simulink model "bike_model_yixiao"  (R2018b)
settings: Solver=FixedStepAuto  StartTime=0.0  StopTime=sim_time  FixedStep=Ts_IMU  MaxStep=Ts  RelTol=1e-3
undefined symbols (not defined in the file): A, A_kalman, B, b_compFilter, B_kalman, b_real, C, C_kalman, complementary, cumulative_dist_along_path, curvature, D, D_kalman, damp, Dead_Band, delay, direct_control, DiscIntNeverNeededParam, Discrete, DX, filter_model, forward_motor_dynamics, fr_oscil, g, gain, I_direct, I_lat, I_steer, IMU_height_model, IMU_height_real, initial_states, initial_x, initial_y, input_velocity, lambda_compFilter, lambda_real, lat_control, look_ahead, lqr_gains, max_handlebar, max_roll, max_steering_motor_acc, max_steering_motor_speed, min_handlebar, min_roll, min_steering_motor_acc, min_steering_motor_speed, Nc, noise, noise_acc, noise_encoder, noise_gyro, noise_hall, noise_pos_meas, Np, osc_roll, osc_steer, P_direct, P_lat, P_steer ... (+20)
libraries: simulink x14, mpclib x2, dspsigops x2, simulink_extras x1, ctrlSharedLib x1
(part 2 of 3)

== system bike_model_yixiao/Reference Position /Reference Position and Angle Selector ==
  total travelled distance : Inport
  1-D Lookup Table : Lookup_n-D  NumberOfTableDimensions=1  BreakpointsForDimension1=cumulative_dist_along_path  Table=path_x  ExtrapMethod=Clip  DiagnosticForOutOfRangeInput=Error  InternalRulePriority=Speed  RndMeth=Simplest  InputSameDT=on
  1-D Lookup Table1 : Lookup_n-D  NumberOfTableDimensions=1  BreakpointsForDimension1=cumulative_dist_along_path  Table=path_y  ExtrapMethod=Clip  DiagnosticForOutOfRangeInput=Error  InternalRulePriority=Speed  RndMeth=Simplest  InputSameDT=on
  Atan2 : Trigonometry  Operator=atan2
  Derivative : Derivative
  Derivative1 : Derivative
  Scope : Scope
  Unwrap : dspsigops/Unwrap  tol=pi  InputProcessing=Columns as channels (frame based)  running=off
  X_sigma : Outport
  Y_sigma : Outport  Port=2
  psi_sigma : Outport  Port=3
  wires:
  total travelled distance/1 -> 1-D Lookup Table1/1, 1-D Lookup Table/1
  Unwrap/1 -> Scope/1, psi_sigma/1
  1-D Lookup Table/1 -> X_sigma/1, Derivative1/1  "interpolated path x value"
  Derivative1/1 -> Atan2/2  "dx"
  Derivative/1 -> Atan2/1  "dy"
  Atan2/1 -> Unwrap/1
  1-D Lookup Table1/1 -> Y_sigma/1, Derivative/1  "interpolated path y value"

== system bike_model_yixiao/Reference Position /Subsystem1 ==
  total travelled distance : Inport
  1-D Lookup Table : Lookup_n-D  NumberOfTableDimensions=1  BreakpointsForDimension1=cumulative_dist_along_path  Table=path_x  ExtrapMethod=Clip  DiagnosticForOutOfRangeInput=Error  InternalRulePriority=Speed  RndMeth=Simplest  InputSameDT=on
  1-D Lookup Table1 : Lookup_n-D  NumberOfTableDimensions=1  BreakpointsForDimension1=cumulative_dist_along_path  Table=path_y  ExtrapMethod=Clip  DiagnosticForOutOfRangeInput=Error  InternalRulePriority=Speed  RndMeth=Simplest  InputSameDT=on
  Atan2 : Trigonometry  Operator=atan2
  Derivative : Derivative
  Derivative1 : Derivative
  Scope : Scope
  Unwrap : dspsigops/Unwrap  tol=pi  InputProcessing=Columns as channels (frame based)  running=off
  X_sigma : Outport
  Y_sigma : Outport  Port=2
  psi_sigma : Outport  Port=3
  wires:
  total travelled distance/1 -> 1-D Lookup Table1/1, 1-D Lookup Table/1
  Unwrap/1 -> Scope/1, psi_sigma/1
  1-D Lookup Table/1 -> X_sigma/1, Derivative1/1  "interpolated path x value"
  Derivative1/1 -> Atan2/2  "dx"
  Derivative/1 -> Atan2/1  "dy"
  Atan2/1 -> Unwrap/1
  1-D Lookup Table1/1 -> Y_sigma/1, Derivative/1  "interpolated path y value"

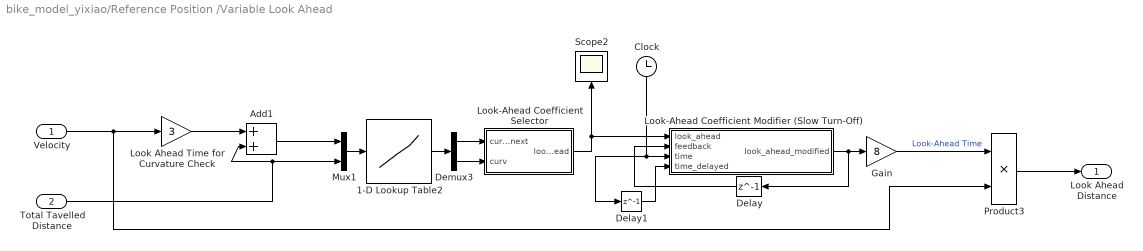
== system bike_model_yixiao/Reference Position /Variable Look Ahead ==
  Velocity : Inport
  Total Tavelled Distance : Inport  Port=2
  1-D Lookup Table2 : Lookup_n-D  NumberOfTableDimensions=1  BreakpointsForDimension1=cumulative_dist_along_path  Table=curvature  ExtrapMethod=Clip  DiagnosticForOutOfRangeInput=Error  InternalRulePriority=Speed  RndMeth=Simplest  InputSameDT=on
  Add1 : Sum
  Clock : Clock
  Delay : Delay  DelayLength=1
  Delay1 : Delay  DelayLength=1
  Demux3 : Demux  Outputs=2
  Gain : Gain  Gain=8
  Look Ahead Time for Curvature Check : Gain  Gain=3
  Look-Ahead Coefficient Selector : MATLAB Function  TreatAsAtomicUnit=on
  "Look-Ahead Coefficient Modifier (Slow Turn-Off) " : MATLAB Function  TreatAsAtomicUnit=on
  Mux1 : Mux  Inputs=2
  Product3 : Product
  Scope2 : Scope
  Look Ahead Distance : Outport
  wires:
  Look Ahead Time for Curvature Check/1 -> Add1/1
  Delay/1 -> "Look-Ahead Coefficient Modifier (Slow Turn-Off) "/2(feedback)
  "Look-Ahead Coefficient Modifier (Slow Turn-Off) "/1(look_ahead_modified) -> Delay/1, Gain/1
  Demux3/1 -> Look-Ahead Coefficient Selector/1(curv_next)
  Look-Ahead Coefficient Selector/1(look_ahead) -> "Look-Ahead Coefficient Modifier (Slow Turn-Off) "/1(look_ahead), Scope2/1
  Clock/1 -> "Look-Ahead Coefficient Modifier (Slow Turn-Off) "/3(time), Delay1/1
  Delay1/1 -> "Look-Ahead Coefficient Modifier (Slow Turn-Off) "/4(time_delayed)
  1-D Lookup Table2/1 -> Demux3/1
  Total Tavelled Distance/1 -> Add1/2, Mux1/2
  Demux3/2 -> Look-Ahead Coefficient Selector/2(curv)
  Gain/1 -> Product3/1  "Look-Ahead Time"
  Add1/1 -> Mux1/1
  Mux1/1 -> 1-D Lookup Table2/1
  Velocity/1 -> Product3/2, Look Ahead Time for Curvature Check/1
  Product3/1 -> Look Ahead Distance/1

== system bike_model_yixiao/Steering Motor/Motor Deadband ==
  Calculated Input : Inport
  Abs : Abs
  Abs1 : Abs
  Constant : Constant  Value=0  SampleTime=Ts
  Constant1 : Constant  Value=0  SampleTime=Ts
  Constant2 : Constant  Value=Dead_Band(2)  SampleTime=Ts
  Constant4 : Constant  Value=Dead_Band(1)  SampleTime=Ts
  Gain : Gain  Gain=-1
  Relay1 : Relay  OnSwitchValue=Dead_Band(3)  OffSwitchValue=-Dead_Band(3)
  Relay2 : Relay  OnSwitchValue=Dead_Band(3)  OffSwitchValue=-Dead_Band(3)
  Sum1 : Sum  Inputs=-+|
  Sum2 : Sum  Inputs=-+|
  Switch : Switch  Criteria=u2 > Threshold
  Switch1 : Switch  Criteria=u2 > Threshold
  Switch2 : Switch  Criteria=u2 > Threshold
  Input Signal After Dead Band : Outport
  wires:
  Constant4/1 -> Sum1/1
  Sum1/1 -> Relay1/1
  Relay1/1 -> Switch/2
  Switch/1 -> Switch1/1
  Constant/1 -> Switch/3
  Switch1/1 -> Input Signal After Dead Band/1
  Switch2/1 -> Switch1/3
  Constant1/1 -> Switch2/3
  Gain/1 -> Sum2/1
  Calculated Input/1 -> Abs/1, Switch2/1, Abs1/1, Switch/1, Switch1/2
  Sum2/1 -> Relay2/1
  Relay2/1 -> Switch2/2
  Abs/1 -> Sum2/2
  Abs1/1 -> Sum1/2
  Constant2/1 -> Gain/1

== system bike_model_yixiao/Steering Motor/Velocity Saturation wrt Max and Min Handle Bar Angles ==
  Reference Steering Rate : Inport
  States : Inport  Port=2
  AND : Logic  IconShape=distinctive  AllPortsSameDT=off  OutDataTypeStr=boolean
  AND1 : Logic  IconShape=distinctive  AllPortsSameDT=off  OutDataTypeStr=boolean
  Compare To Constant : simulink/Logic and Bit Operations/Compare To Constant  relop=>=  const=max_handlebar  OutDataTypeStr=boolean
  Compare To Constant1 : simulink/Logic and Bit Operations/Compare To Constant  relop=<=  const=min_handlebar  OutDataTypeStr=boolean
  Compare To Zero : simulink/Logic and Bit Operations/Compare To Zero  relop=>=  OutDataTypeStr=boolean
  Compare To Zero1 : simulink/Logic and Bit Operations/Compare To Zero  relop=<=  OutDataTypeStr=boolean
  Constant : Constant  Value=0
  Demux : Demux  Outputs=3
  OR : Logic  Operator=OR  IconShape=distinctive  AllPortsSameDT=off  OutDataTypeStr=boolean
  Switch : Switch  Criteria=u2 > Threshold
  Output Steering Rate : Outport
  wires:
  Switch/1 -> Output Steering Rate/1
  Constant/1 -> Switch/1
  States/1 -> Demux/1
  Compare To Constant/1 -> AND/2
  OR/1 -> Switch/2
  Reference Steering Rate/1 -> Switch/3, Compare To Zero/1, Compare To Zero1/1
  Compare To Constant1/1 -> AND1/1
  AND1/1 -> OR/2
  Demux/2 -> Compare To Constant/1, Compare To Constant1/1
  AND/1 -> OR/1
  Compare To Zero1/1 -> AND1/2
  Compare To Zero/1 -> AND/1

== system bike_model_yixiao/Balance Controller/LQR Balancing Control/Balance Controller ==
  Reference Steering Angle : Inport
  Measured Velocity : Inport  Port=2
  Measured States : Inport  Port=3
  LQR Controller : Subsystem  TreatAsAtomicUnit=on  SystemSampleTime=Ts
  Reference States : Subsystem  SystemSampleTime=Ts
  Sum : Sum  Inputs=|+-
  To Workspace : ToWorkspace  VariableName=states_measured  SaveFormat=Timeseries  SampleTime=-1
  Reference Steering Rate : Outport
  wires:
  Reference States/1(Reference States) -> Sum/1
  Sum/1 -> LQR Controller/2(State Error)
  LQR Controller/1(Calculated Input) -> Reference Steering Rate/1
  Reference Steering Angle/1 -> Reference States/2(Delta Ref)
  Measured Velocity/1 -> Reference States/1(Velocity), LQR Controller/1(Velocity)
  Measured States/1 -> To Workspace/1, Sum/2

== system bike_model_yixiao/Balance Controller/MPC attempt 2/Reference States ==
  Velocity : Inport
  Delta Ref : Inport  Port=2
  Bike Parameters : Constant  Value=parameters_real
  Constant : Constant  Value=path_tracking
  Mux5 : Mux  Inputs=3
  Reference Roll Angle Calculator : MATLAB Function  TreatAsAtomicUnit=on
  Switch : Switch  Criteria=u2 > Threshold
  Reference States : Outport
  wires:
  Bike Parameters/1 -> Reference Roll Angle Calculator/1(parameters_real)
  Switch/1 -> Mux5/2, Reference Roll Angle Calculator/3(delta_ref)
  Reference Roll Angle Calculator/1(phi_ref) -> Mux5/1
  Velocity/1 -> Reference Roll Angle Calculator/2(velocity)
  Mux5/1 -> Reference States/1
  Constant/1 -> Switch/2
  Delta Ref/1 -> Switch/1

== system bike_model_yixiao/Complementary filter/Roll Angle Estimation of Accelerometer/Centripetal Acceleration Compensator ==
  Steering Angle : Inport
  Velocity : Inport  Port=2
  Bike Model b : Constant  Value=b_compFilter
  Divide : Product  Inputs=*/
  Gain : Gain  Gain=sin(lambda_compFilter)
  Multiply : Product
  Square : Math  Operator=square  SaturateOnIntegerOverflow=on
  Tan : Trigonometry  Operator=tan
  Estimated Centripetal Acceleration : Outport
  wires:
  Velocity/1 -> Square/1
  Square/1 -> Divide/1
  Bike Model b/1 -> Divide/2
  Steering Angle/1 -> Gain/1
  Divide/1 -> Multiply/1
  Tan/1 -> Multiply/2
  Multiply/1 -> Estimated Centripetal Acceleration/1
  Gain/1 -> Tan/1

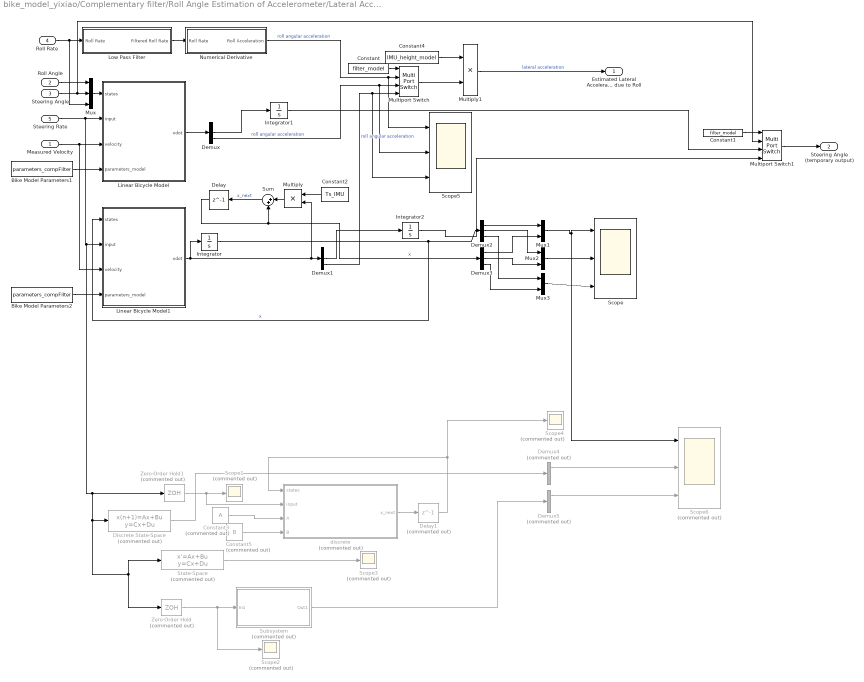
== system bike_model_yixiao/Complementary filter/Roll Angle Estimation of Accelerometer/Lateral Acceleration Compensator ==
  Measured Velocity : Inport
  Roll Angle : Inport  Port=2
  Steering Angle : Inport  Port=3
  Roll Rate : Inport  Port=4
  Steering Rate : Inport  Port=5
  Bike Model Parameters1 : Constant  Value=parameters_compFilter
  Bike Model Parameters2 : Constant  Value=parameters_compFilter
  Constant : Constant  Value=filter_model
  Constant1 : Constant  Value=filter_model
  Constant2 : Constant  Value=Ts_IMU  SampleTime=Ts_IMU
  Constant3 : Constant  Commented=on  Value=A
  Constant4 : Constant  Value=IMU_height_model
  Constant5 : Constant  Commented=on  Value=B
  Delay : Delay  DelayLength=1  InitialCondition=[0 0 0]  SampleTime=Ts_IMU
  Delay1 : Delay  Commented=on  DelayLength=1  InitialCondition=[0 0 0]  SampleTime=Ts_IMU
  Demux{,1..3} (4 alike) : Demux  Outputs=3
  Demux4 : Demux  Commented=on  Outputs=3
  Demux5 : Demux  Commented=on  Outputs=3
  Discrete State-Space : DiscreteStateSpace  Commented=on  A=A  B=B  C=eye(3,3)  D=zeros(3,1)  InitialCondition=[0 0 0]  SampleTime=Ts_IMU
  Integrator : Integrator  InitialCondition=initial_states
  Integrator1 : Integrator  InitialCondition=initial_states(2)
  Integrator2 : Integrator  InitialCondition=initial_states(2)
  Linear Bicycle Model : MATLAB Function  TreatAsAtomicUnit=on
  Linear Bicycle Model1 : MATLAB Function  TreatAsAtomicUnit=on
  Low Pass Filter : Subsystem
  Multiply : Product
  Multiply1 : Product
  Multiport Switch : MultiPortSwitch
  Multiport Switch1 : MultiPortSwitch
  Mux : Mux  Inputs=3
  Mux1 : Mux  Inputs=2
  Mux2 : Mux  Inputs=2
  Mux3 : Mux  Inputs=2
  Numerical Derivative : Subsystem
  Scope : Scope  NumInputPorts=3
  Scope{1..4} (4 alike) : Scope  Commented=on
  Scope5 : Scope  NumInputPorts=3
  Scope6 : Scope  Commented=on  NumInputPorts=3
  State-Space : StateSpace  Commented=on  A=sys_con.A  B=sys_con.B  C=eye(3,3)  D=zeros(3,1)  InitialCondition=[0 0 0]
  Subsystem : Subsystem  Commented=on  TreatAsAtomicUnit=on  SystemSampleTime=Ts_IMU
  Sum : Sum  Inputs=|++
  Zero-Order Hold : ZeroOrderHold  Commented=on  SampleTime=Ts_IMU
  Zero-Order Hold1 : ZeroOrderHold  Commented=on  SampleTime=Ts_IMU
  discrete : MATLAB Function  Commented=on  TreatAsAtomicUnit=on
  Estimated Lateral Accelerattion due to Roll : Outport
  Steering Angle (temporary output) : Outport  Port=2
  wires:
  Numerical Derivative/1(Roll Acceleration) -> Scope5/1, Multiport Switch/2  "roll angular acceleration"
  Roll Rate/1 -> Mux/3, Low Pass Filter/1(Roll Rate)
  Constant4/1 -> Multiply1/1
  Multiply1/1 -> Estimated Lateral Accelerattion due to Roll/1  "lateral acceleration"
  Low Pass Filter/1(Filtered Roll Rate) -> Numerical Derivative/1(Roll Rate)
  Linear Bicycle Model/1(xdot) -> Demux/1
  Demux/3 -> Scope5/2, Multiport Switch/3  "roll angular acceleration"
  Bike Model Parameters1/1 -> Linear Bicycle Model/4(parameters_model)
  Measured Velocity/1 -> Linear Bicycle Model1/3(velocity), Linear Bicycle Model/3(velocity)
  Mux/1 -> Linear Bicycle Model/1(states)
  Roll Angle/1 -> Mux/1
  Steering Angle/1 -> Multiport Switch1/2, Mux/2
  Constant/1 -> Multiport Switch/1
  Multiport Switch/1 -> Multiply1/2
  Demux1/3 -> Scope5/3, Multiport Switch/4  "roll angular acceleration"
  Bike Model Parameters2/1 -> Linear Bicycle Model1/4(parameters_model)
  Delay/1 -> Demux3/1, Sum/2  "x"
  Multiply/1 -> Sum/1
  Constant2/1 -> Multiply/1
  Integrator/1 -> Linear Bicycle Model1/1(states), Demux2/1  "x"
  Demux2/1 -> Mux1/1
  Demux3/1 -> Mux1/2
  Demux2/2 -> Mux2/1
  Demux3/2 -> Mux2/2
  Demux2/3 -> Mux3/1
  Demux3/3 -> Mux3/2
  Mux2/1 -> Scope/2
  Mux1/1 -> Scope6/1, Scope/1
  Mux3/1 -> Scope/3
  Linear Bicycle Model1/1(xdot) -> Multiply/2, Demux1/1, Integrator/1
  State-Space/1 -> Scope3/1
  Delay1/1 -> Scope4/1, discrete/1(states)
  Zero-Order Hold/1 -> Scope2/1, Subsystem/1(In1)
  discrete/1(x_next) -> Delay1/1
  Constant5/1 -> discrete/4(B)
  Constant3/1 -> discrete/3(A)
  Sum/1 -> Delay/1  "x_next"
  Zero-Order Hold1/1 -> discrete/2(input), Scope1/1
  Multiport Switch1/1 -> Steering Angle (temporary output)/1
  Constant1/1 -> Multiport Switch1/1
  Steering Rate/1 -> Zero-Order Hold/1, State-Space/1, Discrete State-Space/1, Zero-Order Hold1/1, Linear Bicycle Model1/2(input), Linear Bicycle Model/2(input)
  Integrator1/1 -> Multiport Switch1/3
  Demux/2 -> Integrator1/1
  Demux1/2 -> Integrator2/1
  Integrator2/1 -> Multiport Switch1/4
  Demux4/1 -> Scope6/2
  Demux5/1 -> Scope6/3
  Discrete State-Space/1 -> Demux4/1
  Subsystem/1(Out1) -> Demux5/1

== system bike_model_yixiao/Physical Bike/Global Angles and Coordinates Calculator - Position/Measured Bike Angles to Global Angles ==
  Velocity : Inport
  Measured Steering Angle : Inport  Port=2
  " Bike Parameters Model " : Constant  Value=parameters_compFilter
  Integrator : Integrator
  MATLAB Function : MATLAB Function  TreatAsAtomicUnit=on
  To Workspace6 : ToWorkspace  VariableName=PSI  SaveFormat=Timeseries  SampleTime=Ts
  To Workspace7 : ToWorkspace  VariableName=BETA  SaveFormat=Timeseries  SampleTime=Ts
  Psi : Outport
  Beta : Outport  Port=2
  wires:
  MATLAB Function/2(beta) -> Beta/1, To Workspace7/1
  MATLAB Function/1(psi_d) -> Integrator/1
  Integrator/1 -> Psi/1, To Workspace6/1
  " Bike Parameters Model "/1 -> MATLAB Function/2(parameters_model)
  Measured Steering Angle/1 -> MATLAB Function/3(delta)
  Velocity/1 -> MATLAB Function/1(v)

== system bike_model_yixiao/Physical Bike/Global Angles and Coordinates Calculator - Position/Measured Global Angles to Global Coordinates ==
  Velocity : Inport
  Psi : Inport  Port=2
  Beta : Inport  Port=3
  Constant : Constant  Value=initial_y
  Constant1 : Constant  Value=initial_x
  Integrator1 : Integrator
  Integrator2 : Integrator
  MATLAB Function1 : MATLAB Function  TreatAsAtomicUnit=on
  Mux : Mux  Inputs=2
  Sum : Sum  Inputs=|++
  Sum1 : Sum  Inputs=++|
  "Position (X, Y)" : Outport
  wires:
  MATLAB Function1/2(Ydot) -> Integrator2/1  "Ydot"
  MATLAB Function1/1(Xdot) -> Integrator1/1  "Xdot"
  Psi/1 -> MATLAB Function1/2(psi)
  Beta/1 -> MATLAB Function1/3(beta)
  Velocity/1 -> MATLAB Function1/1(v)
  Integrator2/1 -> Sum/1
  Constant/1 -> Sum/2
  Sum/1 -> Mux/2
  Integrator1/1 -> Sum1/2
  Sum1/1 -> Mux/1
  Constant1/1 -> Sum1/1
  Mux/1 -> "Position (X, Y)"/1

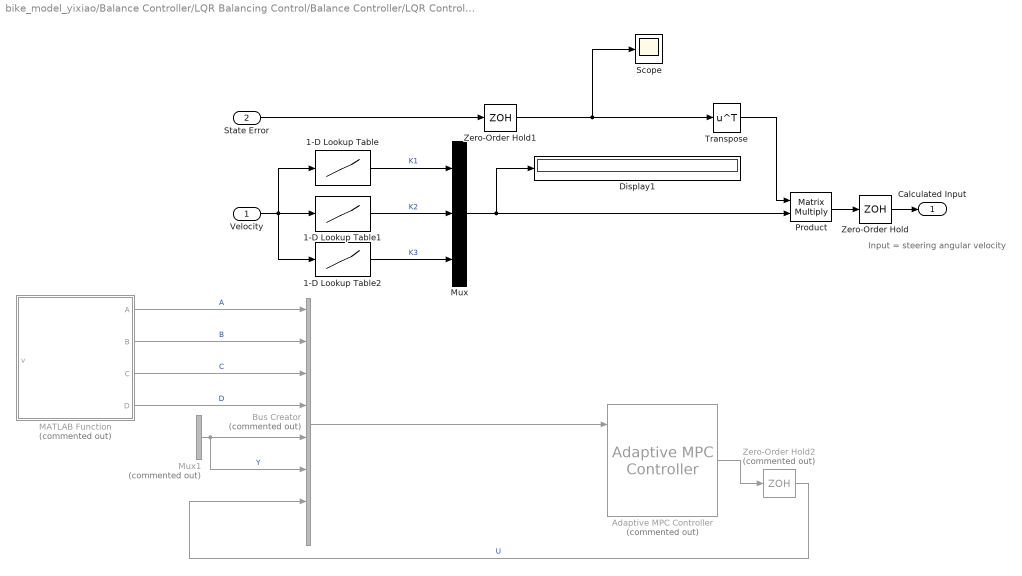
== system bike_model_yixiao/Balance Controller/LQR Balancing Control/Balance Controller/LQR Controller ==
  note: Input = steering angular velocity
  Velocity : Inport
  State Error : Inport  Port=2
  1-D Lookup Table : Lookup_n-D  NumberOfTableDimensions=1  BreakpointsForDimension1=velocity_lqr  BreakpointsForDimension2=velocity_lqr  BreakpointsForDimension3=velocity_lqr  BreakpointsForDimension4=velocity_lqr  Table=lqr_gains(:,1)  InternalRulePriority=Speed  RndMeth=Simplest  InputSameDT=on
  1-D Lookup Table1 : Lookup_n-D  NumberOfTableDimensions=1  BreakpointsForDimension1=velocity_lqr  BreakpointsForDimension2=velocity_lqr  BreakpointsForDimension3=velocity_lqr  BreakpointsForDimension4=velocity_lqr  Table=lqr_gains(:,2)  InternalRulePriority=Speed  RndMeth=Simplest  InputSameDT=on
  1-D Lookup Table2 : Lookup_n-D  NumberOfTableDimensions=1  BreakpointsForDimension1=velocity_lqr  BreakpointsForDimension2=velocity_lqr  BreakpointsForDimension3=velocity_lqr  BreakpointsForDimension4=velocity_lqr  Table=lqr_gains(:,3)  InternalRulePriority=Speed  RndMeth=Simplest  InputSameDT=on
  Adaptive MPC Controller : mpclib/Adaptive MPC Controller  Commented=on  SCDEnableBlockLinearizationSpecification=on  enable_value=0  updateMPCinCallerWorkspace=on  md_inport=off  mv_inport=off  return_cost=off  return_mvseq=off  return_qpstatus=off  return_xseq=off  return_state=off  return_ovseq=off  state_inport=off  isltv_plant=off  umin_inport=off  umax_inport=off  ymin_inport=off  ymax_inport=off  cc_inport=off  ywt_inport=off  uwt_inport=off  duwt_inport=off  rhoeps_inport=off  uref_inport=off  BlockDataType=double  SampleTimeInherited=off  switch_inport=off
      settings: SourceProductName=Model Predictive Control Toolbox
  Bus Creator : BusCreator  Commented=on  Inputs=A,B,C,D,X,Y,U,DX
  Display1 : Display
  MATLAB Function : MATLAB Function  Commented=on  TreatAsAtomicUnit=on
  Mux : Mux  Inputs=3
  Mux1 : Mux  Commented=on  Inputs=3
  Product : Product  Multiplication=Matrix(*)
  Scope : Scope
  Transpose : Math  Operator=transpose  SaturateOnIntegerOverflow=on
  Zero-Order Hold : ZeroOrderHold  SampleTime=Ts
  Zero-Order Hold1 : ZeroOrderHold  SampleTime=Ts
  Zero-Order Hold2 : ZeroOrderHold  Commented=on  SampleTime=-1
  Calculated Input : Outport
  wires:
  1-D Lookup Table/1 -> Mux/1  "K1"
  1-D Lookup Table1/1 -> Mux/2  "K2"
  State Error/1 -> Zero-Order Hold1/1
  Product/1 -> Zero-Order Hold/1
  1-D Lookup Table2/1 -> Mux/3  "K3"
  Velocity/1 -> 1-D Lookup Table2/1, 1-D Lookup Table1/1, 1-D Lookup Table/1
  Mux/1 -> Product/2, Display1/1
  Transpose/1 -> Product/1
  Zero-Order Hold/1 -> Calculated Input/1
  Zero-Order Hold1/1 -> Scope/1, Transpose/1
  MATLAB Function/1(A) -> Bus Creator/1  "A"
  MATLAB Function/2(B) -> Bus Creator/2  "B"
  MATLAB Function/3(C) -> Bus Creator/3  "C"
  MATLAB Function/4(D) -> Bus Creator/4  "D"
  Bus Creator/1 -> Adaptive MPC Controller/1
  Mux1/1 -> Bus Creator/6, Bus Creator/5  "Y"
  Adaptive MPC Controller/1 -> Zero-Order Hold2/1
  Zero-Order Hold2/1 -> Bus Creator/7  "U"

== system bike_model_yixiao/Balance Controller/LQR Balancing Control/Balance Controller/Reference States ==
  Velocity : Inport
  Delta Ref : Inport  Port=2
  Bike Parameters : Constant  Value=parameters_real
  Constant : Constant  Value=path_tracking
  Mux5 : Mux  Inputs=3
  Reference Roll Angle Calculator : MATLAB Function  TreatAsAtomicUnit=on
  Switch : Switch  Criteria=u2 > Threshold
  Reference States : Outport
  wires:
  Bike Parameters/1 -> Reference Roll Angle Calculator/1(parameters_real)
  Switch/1 -> Mux5/2, Reference Roll Angle Calculator/3(delta_ref)
  Reference Roll Angle Calculator/1(phi_ref) -> Mux5/1
  Velocity/1 -> Reference Roll Angle Calculator/2(velocity)
  Mux5/1 -> Reference States/1
  Constant/1 -> Switch/2
  Delta Ref/1 -> Switch/1

== system bike_model_yixiao/Complementary filter/Roll Angle Estimation of Accelerometer/Lateral Acceleration Compensator/Low Pass Filter ==
  Roll Rate : Inport
  Delay18 : Delay  DelayLength=1
  Gain4 : Gain  Gain=roll_rate_coef
  Gain6 : Gain  Gain=1-roll_rate_coef
  Scope7 : Scope  NumInputPorts=2
  Sum4 : Sum  Inputs=|++
  Filtered Roll Rate : Outport
  wires:
  Gain6/1 -> Sum4/1
  Gain4/1 -> Sum4/2
  Sum4/1 -> Filtered Roll Rate/1, Delay18/1, Scope7/2  "Filtered Roll Rate"
  Delay18/1 -> Gain4/1
  Roll Rate/1 -> Scope7/1, Gain6/1  "Measured Roll Rate"

== system bike_model_yixiao/Complementary filter/Roll Angle Estimation of Accelerometer/Lateral Acceleration Compensator/Numerical Derivative ==
  Roll Rate : Inport
  Delay18 : Delay  DelayLength=1
  Gain3 : Gain  Gain=1/Ts_IMU
  Sum3 : Sum  Inputs=|+-
  Roll Acceleration : Outport
  wires:
  Sum3/1 -> Gain3/1
  Delay18/1 -> Sum3/2
  Roll Rate/1 -> Sum3/1, Delay18/1
  Gain3/1 -> Roll Acceleration/1

== system bike_model_yixiao/Complementary filter/Roll Angle Estimation of Accelerometer/Lateral Acceleration Compensator/Subsystem ==
  In1 : Inport
  Constant : Constant  Value=A
  Constant1 : Constant  Value=B
  Delay1 : Delay  DelayLength=1  InitialCondition=[0 0 0]  SampleTime=Ts_IMU
  Multiply : Product  Multiplication=Matrix(*)
  Multiply1 : Product  Multiplication=Matrix(*)
  Sum2 : Sum  Inputs=|++
  Out1 : Outport
  wires:
  Sum2/1 -> Delay1/1
  Multiply1/1 -> Sum2/2
  In1/1 -> Multiply1/2  "u"
  Delay1/1 -> Multiply/2, Out1/1  "x"
  Multiply/1 -> Sum2/1
  Constant/1 -> Multiply/1
  Constant1/1 -> Multiply1/1

== matlab function bike_model_yixiao/Balance Controller/LQR Balancing Control/Balance Controller/Reference States/Reference Roll Angle Calculator ==
  data: parameters_real input; velocity input; delta_ref input; phi_ref output
function phi_ref = fcn(parameters_real, velocity, delta_ref)
g = parameters_real(1);
b = parameters_real(3);
v = velocity;

phi_ref = -atan(v^2 / (g * b) * delta_ref); % tan(theta_ref));

== matlab function bike_model_yixiao/Physical Bike/Linear Bicycle Model ==
  data: states input; input input; xdot output; velocity input; disturbance input; parameters_real input; parameters_f_b_real input
function xdot = fcn(states,input,velocity,disturbance,parameters_real,parameters_f_b_real)

delta_d=input;
v=velocity;
d1=disturbance(1);
d2=disturbance(2);
d3=disturbance(3);

% 1=frame | 2=box
m1=parameters_f_b_real(1);
m2=parameters_f_b_real(2);
h1=parameters_f_b_real(3);
h2=parameters_f_b_real(4);
a1=parameters_f_b_real(5);
a2=parameters_f_b_real(6);
c1=parameters_f_b_real(7);
c2=parameters_f_b_real(8);
b1=parameters_f_b_real(9);
b2=parameters_f_b_real(10);
l1=parameters_f_b_real(11);
l2=parameters_f_b_real(12);

g=parameters_real(1);
%h=parameters_real(2);
b=parameters_real(3);
%a=parameters_real(4);
lambda=parameters_real(5);
c=parameters_real(6);

phi=states(1);
delta=states(2);
phi_d=states(3);

A=((m1/12)*((c1^2)+(b1^2)))+(m1*(h1^2))+((m2/12)*((c2^2)+(b2^2)))+(m2*(h2^2));
B=((m1/12)*((l1^2)+(b1^2)))-(m1*a1*h1)+((m2/12)*((c2^2)+(b2^2)))+(m2*a2*h2);
D=(((m1*h1)+(m2*h2))*(v^2))-(c*g*((m1*a1)-(m2*a2)));

xdot1=phi_d+d1;
xdot2=delta_d+d2;
xdot3=((((m1*h1)+(m2*h2))*g)/A)*phi+((D*sin(lambda))/(b*A))*delta+d3+((B*v*sin(lambda))/(b*A))*delta_d;

xdot=[xdot1 xdot2 xdot3];

== matlab function bike_model_yixiao/Balance Controller/LQR Balancing Control/Balance Controller/LQR Controller/MATLAB Function ==
  data: v input; A output; B output; C output; D output
function [A, B, C, D] = sys_linearization(v)
persistent h_real b_real c_real lambda_real a_real g Ts
% Real Bike Parameters
% Global system (frame+box as 1 volume)
if isempty(h_real)
    h_real = 0.48;             % height of center of mass [m]
    b_real = 1.095;            % length between wheel centers [m]
    c_real = 0.06;             % length between front wheel contact point and the 
    lambda_real = deg2rad(70); % angle of the fork axis [deg]
    a_real = 0.34;             % b_real-0.77;
    g = 9.81;                  % gravity [m/s^2]
    Ts = 0.04;
end

A_m = [0      0            1;
       0      0            0;
       g/h_real    sin(lambda_real)*(h_real*v^2-g*a_real*c_real)/(h_real^2*b_real)   0];
B_m = [0; 1; (a_real*v*sin(lambda_real))/(h_real*b_real)];
C_m = eye(3);
D_m = zeros(3,1);
sys_con = ss(A_m,B_m,C_m,D_m);
sys_dis = c2d(sys_con,Ts);

A = sys_dis.A;
B = sys_dis.B;
C = sys_dis.C;
D = sys_dis.D;

    
end

== matlab function bike_model_yixiao/Reference Position /Variable Look Ahead/Look-Ahead Coefficient Modifier (Slow Turn-Off)  ==
  data: look_ahead input; look_ahead_modified output; feedback input; time input; time_delayed input
function look_ahead_modified = fcn(look_ahead, feedback, time, time_delayed)

step=time-time_delayed;

kill_time=3;

delta=(feedback*step)/kill_time;

if look_ahead-feedback<-0.0001
    look_ahead_modified=feedback-delta;
else
    look_ahead_modified = look_ahead;
end
    

end

== matlab function bike_model_yixiao/Balance Controller/MPC Control/MATLAB Function ==
  data: v input; A output; B output; C output; D output
function [A, B, C, D] = sys_linearization(v)
persistent h_real b_real c_real lambda_real a_real g Ts
% Real Bike Parameters
% Global system (frame+box as 1 volume)
if isempty(h_real)
    h_real = 0.48;             % height of center of mass [m]
    b_real = 1.095;            % length between wheel centers [m]
    c_real = 0.06;             % length between front wheel contact point and the 
    lambda_real = deg2rad(70); % angle of the fork axis [deg]
    a_real = 0.34;             % b_real-0.77;
    g = 9.81;                  % gravity [m/s^2]
    Ts = 0.04;
end

A_m = [0      0            1;
       0      0            0;
       g/h_real    sin(lambda_real)*(h_real*v^2-g*a_real*c_real)/(h_real^2*b_real)   0];
B_m = [0; 1; (a_real*v*sin(lambda_real))/(h_real*b_real)];
C_m = eye(3);
D_m = zeros(3,1);
sys_con = ss(A_m,B_m,C_m,D_m);
sys_dis = c2d(sys_con,Ts);

A = sys_dis.A;
B = sys_dis.B;
C = sys_dis.C;
D = sys_dis.D;

    
end

== matlab function bike_model_yixiao/Reference Position /Variable Look Ahead/Look-Ahead Coefficient Selector ==
  data: curv_next input; look_ahead output; curv input
function look_ahead = fcn(curv_next, curv)


if curv>-0.01 && curv<0.01
    curv=0;
end

if curv_next>-0.01 && curv_next<0.01
    curv_next=0;
end



if curv>=0
    if curv-curv_next>0
        look_ahead=0;
    else
        look_ahead=curv_next-curv;
    end
else
    if curv-curv_next<0
        look_ahead=0;
    else
        look_ahead=curv-curv_next;
    end
end



end

== matlab function bike_model_yixiao/Complementary filter/Roll Angle Estimation of Accelerometer/Lateral Acceleration Compensator/Linear Bicycle Model ==
  data: states input; input input; xdot output; velocity input; parameters_model input
function xdot = fcn(states,input,velocity,parameters_model)

delta_d=input;
v=velocity;

g=parameters_model(1);
h=parameters_model(2);
b=parameters_model(3);
a=parameters_model(4);
lambda=parameters_model(5);
c=parameters_model(6);

phi=states(1);
delta=states(2);
phi_d=states(3);

xdot1=phi_d;
xdot2=delta_d;
xdot3=(g/h)*phi+((a*v)/(b*h))*sin(lambda)*delta_d+((h*v^2-g*a*c)/(b*h^2))*sin(lambda)*delta;

xdot=[xdot1 xdot2 xdot3];

== matlab function bike_model_yixiao/Physical Bike/Global Angles and Coordinates Calculator - Position/Measured Bike Angles to Global Angles/MATLAB Function ==
  data: v input; parameters_model input; delta input; psi_d output; beta output
function [psi_d, beta]  = fcn(v, parameters_model, delta)

b = parameters_model(3);
a = parameters_model(4);

beta = atan((a / (b)) * tan(delta));
psi_d = (v / a) * sin(beta);

== matlab function bike_model_yixiao/Balance Controller/MPC attempt 2/MATLAB Function ==
  data: x0 input; u output; eta output; xk0 input; u0 input; Nc input; Np input; r input; Delta_t input; xk output; v input
function [u,eta,xk] =  MPC_LQR_PosVel_solve(x0,xk0,u0,Nc,Np,r,Delta_t,v)
% This Function export the Optimal MPC estimation based on the states
% It runs at timestep k (so now),calculate the signal input for next timestep.
% % % % % % % % % % % % % % % % % % % % % % % % % % % % % % % % % % % % % % 
% 
% Input: 
% -> x0 := The current(k_{th} step) states column (state-space model), includes
% [x0;y0;Psi0;u;v;w;]
% -> xk0 := The Augmented System states, includes [\delta x_m(k); y(k)]
% -> Nc := The control horizon, which means, take actions(manipulate the
% input signal in the next Nc steps)
% -> Np := Prediction Horizon,estimate the states in the next Np steps;ß
% -> r := The reference signal, indicating which states you want to
% achieve,[x_d;y_d;Psi_d;u_d;v_d;w_d;]; 
% -> Delta_t := The sample time for discritization
% % % % % % % % % % % % % % % % % % % % % % % % % % % % % % % % % % % % % % 
% 
% Output:
% -> eta := The optimal \delta U input signal for the system in next Nc Steps,
% [\delta_TauX1;\delta_TauY1;\delta_TauPsi1;\delta_TauX2;\delta_TauY2;...;TauXNc;TauYNc;TauPsiNc];
% -> xk  := The estimation of xk,which may be used for comparison how good
% it tracks the trajectory
 
%% Initialization





% u = zeros(3,1);



%%
[A_m,B_m] = Lin_Sys(v);

C_m = eye(3);
D_m = zeros(3,1);
% The Input Increment Setting

R_bar = zeros(Nc*3);
Wr = 1e3;  % The Multipiler for Increment Input
coder.extrinsic('sqrt')
Kx_gain = 0;
Ky_gain = 0;
Kx_gain = sqrt((x0(1)-r(1))^2); % When it is going to reach the target, Vel is important
Ky_gain = sqrt((x0(2)-r(2))^2);
Yaw_gain = 0;
Yaw_gain = sqrt((x0(3)-r(3))^2 );

% The Input Weight setting
% 
K_u      = 1e-6*eye(Nc,Nc);
for i = 1:Nc
   K_u(i,i) = 1e-10;
end

K_bar = zeros(Np*3);
for i = 1:Np
   K_bar((3)*i-2,(3)*i-2) = 1e4./(1e-2*Kx_gain+1e-3); % The Weight for \Phi
   K_bar((3)*i-1,(3)*i-1) = 1e4./(1e-2*Ky_gain+1e-3); % The Weight for Steering \delta
   K_bar((3)*i,(3)*i)     = 1e7./(1e-2*Yaw_gain+1e-3); % The Weight for \dot{\Phi}
end

K_bar((3)*i-2,(3)*i-2) = 10*K_bar((3)*i-2,(3)*i-2) ; % The terminal weight for \Phi
K_bar((3)*i-1,(3)*i-1) = 10*K_bar((3)*i-1,(3)*i-1) ; % The Terminal Weight for Steering \delta
K_bar((3)*i,(3)*i)     = 1000*K_bar((3)*i,(3)*i) ;  % The Terminal Weight for \dot{\Phi}
% Rs = ones(Np,3)*r;

% MagSurge = 400*1e4;
% MagSway  = 100*1e4;
% MagYaw   = 1e6*1e4;
% DeltaSurge = 5e4;
% DeltaSway  = 5e4;
% DeltaYaw   = 5e7;
% 
% MagSurge = 100*1e4;
% MagSway  = 100*1e4;
% MagYaw   = 1e6*1e4;
% DeltaSurge = 5e4;
% DeltaSway  = 5e4;
% DeltaYaw   = 5e7;
% MagSurge = 1e4;
% MagSway  = 1e4;
% MagYaw   = 1e4;
% 
% end


%% Discretization
coder.extrinsic('c2dm','sum');

[Ap,Bp,Cp,~]=c2dm(A_m,B_m,C_m,D_m,Delta_t,'zoh');

%% Augumented System 
[Phi_Phi,Phi_F,Phi_R,A_e,B_e,~,~,~] = mpcgain(Ap,Bp,Cp,Nc,Np,r,K_bar);


%% solve the optimization problem

% H0 = 2*(Phi_Phi + R_bar); % 3*Nc by 3*Nc
% f0 = -2*(Phi_R-Phi_F*xk0); % 3*Nc by 1
% 
% 
% % The Positive Part for Manipulated Variable(Input) Constraints
% A_cons1 = eye(3*Nc,3*Nc);
% B_cons1 = zeros(3*Nc,1);
% for j = 1:Nc % The #column
%     for i = 1+j:Nc % The #row 
%     A_cons1(3*i-2:3*i,3*j-2:3*j) = eye(3);
% %     A_cons(3*(Nc+i)-2:3*(Nc+i),3*j-2:3*j) = -eye(3);
%     end
%     B_cons1(3*j-2:3*j,1) = [MagSurge;MagSway;MagYaw]-u0;
% %     B_cons(3*(Nc+i)-2:3*(Nc+i),1) =[10000*1e4;10000*1e4;1e4*1e5]+u0;
% end
% 
% % The Negative Part for Manipulated Variable(Input) Constraints
% A_cons2 = eye(3*Nc,3*Nc);
% B_cons2 = zeros(3*Nc,1);
% 
% for j = 1:Nc % The #column
%     for i = 1+j:Nc % The #row 
%     A_cons2(3*i-2:3*i,3*j-2:3*j) = -eye(3);
% %     A_cons2(3*(Nc+i)-2:3*(Nc+i),3*j-2:3*j) = -eye(3);
%     end
%     B_cons2(3*j-2:3*j,1) = [MagSurge;MagSway;MagYaw]+u0;
% %     B_cons2(3*(Nc+i)-2:3*(Nc+i),1) =[10000*1e4;10000*1e4;1e4*1e5]+u0;
% end
% 
% % The Constraints for Input Increment Positive Part
% 
% A_cons3 = eye(3*Nc,3*Nc);
% B_cons3 = zeros(3*Nc,1);
% 
% Wr = 1e3;  % The Multipiler for Increment Input
% 
% for i = 1:Nc % The #row
%     B_cons3(3*i-2:3*i,1) = [DeltaSurge;DeltaSway;DeltaYaw]*Wr;
% end
% 
% % The Constraints for Input Increment Negative Part
% 
% A_cons4 = -eye(3*Nc,3*Nc);
% B_cons4 = zeros(3*Nc,1);
% 
% for i = 1:Nc % The #row
%     B_cons4(3*i-2:3*i,1) = [DeltaSurge;DeltaSway;DeltaYaw]*Wr;
% end


% Constructing the 3Nc*3Nc Lower-Diagnol Identity Matrix P:
%      1     0     0     0     0     0     
%      0     1     0     0     0     0     
%      0     0     1     0     0     0     
%      1     0     0     1     0     0     
%      0     1     0     0     1     0     
%      0     0     1     0     0     1 3Nc*3Nc This is also useful for
%      constrainting the input U

% % The Input sequence as 
% % [ u0;u0;...]Nc*1
P = eye(Nc,Nc);
U0= zeros(Nc,1);
% 
% A_cons1 = zeros(Nc,Nc);
% B_cons1 = zeros(Nc,1);
% A_cons2 = zeros(Nc,Nc);
% B_cons2 = zeros(Nc,1);
% A_cons3 = eye(Nc,Nc);
% B_cons3 = zeros(Nc,1);
% A_cons4 = -eye(Nc,Nc);
% B_cons4 = zeros(Nc,1);
% 
% 
for j = 1:Nc % The #column
    for i = 1+j:Nc % The #row 
    P(i,j) = 1;
    end
    U0(j) = u0;
%     B_cons1(3*j-2:3*j,1) = [MagSurge;MagSway;MagYaw]-u0;
%     B_cons2(3*j-2:3*j,1) = [MagSurge;MagSway;MagYaw]+u0;
%     B_cons3(3*j-2:3*j,1) = [DeltaSurge;DeltaSway;DeltaYaw]*Wr;
end
% B_cons4 = B_cons3;
% A_cons1 = P;
% A_cons2 = -P;



H0 = 2*(Phi_Phi + R_bar+P.'*K_u*P); % Nc by Nc
f0 = 2*(-Phi_R+Phi_F*xk0+P.'*K_u*U0); % Nc by 1

% 
% A_cons = [A_cons1;A_cons2;A_cons3;A_cons4];
% B_cons = [B_cons1;B_cons2;B_cons3;B_cons4];
% 
% 
% A_cons = [A_cons1;A_cons2;];
% B_cons = [B_cons1;B_cons2;];

% B_cons1 = double(B_cons1);
x=-H0\f0; % Calculate an Optimal Solution WITHOUT CONSTRAINTS
% x = QPhild(H0,f0,A_cons,B_cons);
% size(B_e)
% [x,fval] = quadprog(H0,f0,[],[],[],[]);
% [x,fval] = quadprog(H0,f0,A_cons,B_cons,A_Eq1,B_Eq1);
% coder.extrinsic('quadprog');
% x = quadprog(H0,f0,A_cons,B_cons);
eta = x(1); % The force increments to be applied
u = u0 + eta;
% xk = zeros(6,1);
xk = A_e*xk0 + B_e*eta;

end



function [A_m B_m] = Lin_Sys(v)

% % % % % % % % % % % % % % % % % % % % % % % % % % % % % % % % % % % 
% 3-DOF Ship model Linearization
% 
% Input:
% v : rear wheel velocity
%
% Output:
% A 3*3 Linearized System Matrix for \dot{x} = A x + B u
% B 3*1 The Coefficient Matrix for input u
% 
% 
% 
% state x:= [ \Phi \delta \dot{\Phi} ]
% % % % % % % % % % % % % % % % % % % % % % % % % % % % % % % % % % % 

persistent h_real b_real c_real lambda_real a_real g 
% Real Bike Parameters
% Global system (frame+box as 1 volume)
if isempty(h_real)
    h_real = 0.48;             % height of center of mass [m]
    b_real = 1.095;            % length between wheel centers [m]
    c_real = 0.06;             % length between front wheel contact point and the 
    lambda_real = deg2rad(70); % angle of the fork axis [deg]
    a_real = 0.34;             % b_real-0.77;
    g = 9.81;                  % gravity [m/s^2]
end

A_m = [0      0            1;
       0      0            0;
       g/h_real    sin(lambda_real)*(h_real*v^2-g*a_real*c_real)/(h_real^2*b_real)   0];
B_m = [0; 1; (a_real*v*sin(lambda_real))/(h_real*b_real)];
C_m = eye(3);
D_m = zeros(3,1);

end
 
function [Phi_Phi,Phi_F,Phi_R,A_e, B_e,C_e,F,Phi] = mpcgain(Ap,Bp,Cp,Nc,Np,r,K_bar)

% coder.extrinsic('size','eye','zeros');
% coder.varsize('m1',[]   );
m1=size(Cp,1);
[n1,n_in]=size(Bp);
A_e=eye(n1+m1,n1+m1);
A_e(1:n1,1:n1)=Ap;
A_e(n1+1:n1+m1,1:n1)=Cp*Ap;
B_e=zeros(n1+m1,n_in);
B_e(1:n1,:)=Bp;
B_e(n1+1:n1+m1,:)=Cp*Bp;
C_e=zeros(m1,n1+m1);
C_e(:,n1+1:n1+m1)=eye(m1,m1);
[wid,~] = size(C_e);
h = zeros(6*Np,12);
F = zeros(6*Np,12);
h(1:wid,:)=C_e;
F(1:wid,:)=C_e*A_e;

for kk=2:Np
h((kk-1)*wid+1:kk*wid,:)=h((kk-2)*wid+1:(kk-1)*wid,:)*A_e;
F((kk-1)*wid+1:kk*wid,:)= F((kk-2)*wid+1:(kk-1)*wid,:)*A_e;
end

v=h*B_e;

len1 = size(B_e,2);
Phi=zeros(Np*wid,Nc*len1); %declare the dimension of Phi

Phi(:,1:len1)=v; % first column of Phi
% len1 = wid; % the length for CB,CAB,...
for i=2:Nc
    Phi(:,(i-1)*len1+1:i*len1)=[zeros((i-1)*wid,len1);v(1:(Np-i+1)*wid,1:len1)]; %Toeplitz matrix
end

BarRs = zeros(Np*wid,1);

    for i = 1:Np
        BarRs((i-1)*wid+1:i*wid,1) = r;
    end

% BarRs
Phi_Phi = Phi.'*K_bar*Phi;
Phi_Phi = (Phi_Phi.' + Phi_Phi)/2;
% F
Phi_F= Phi'*K_bar*F;
Phi_R=Phi.'*K_bar*BarRs;


end

== matlab function bike_model_yixiao/Physical Bike/Nonlinear Bicycle Model ==
  data: states input; input input; xdot output; velocity input; disturbance input; parameters_real input; parameters_f_b_real input
function xdot = fcn(states,input,velocity,disturbance,parameters_real,parameters_f_b_real)

delta_d=input;
v=velocity;
d1=disturbance(1);
d2=disturbance(2);
d3=disturbance(3);

% 1=frame | 2=box
m1=parameters_f_b_real(1);
m2=parameters_f_b_real(2);
h1=parameters_f_b_real(3);
h2=parameters_f_b_real(4);
a1=parameters_f_b_real(5);
a2=parameters_f_b_real(6);
c1=parameters_f_b_real(7);
c2=parameters_f_b_real(8);
b1=parameters_f_b_real(9);
b2=parameters_f_b_real(10);
l1=parameters_f_b_real(11);
l2=parameters_f_b_real(12);
if length(parameters_f_b_real) > 12
    m3=parameters_f_b_real(13);
    d =parameters_f_b_real(14);
else
    m3 = 0;
    d = 0;
end

g=parameters_real(1);
%h=parameters_real(2);
b=parameters_real(3);
%a=parameters_real(4);
lambda=parameters_real(5);
c=parameters_real(6);

A=((m1/12)*((c1^2)+(b1^2)))+(m1*(h1^2))+((m2/12)*((c2^2)+(b2^2)))+(m2*(h2^2));
B=(m1*a1*h1)-(m2*a2*h2);
D=(((m1*h1)+(m2*h2))*(v^2))-(c*g*((m1*a1)-(m2*a2)));

phi=states(1);
delta=states(2);
phi_d=states(3);
 
xdot1=phi_d+d1;
xdot2=delta_d+d2;
xdot3=((((m1*h1)+(m2*h2))*g)*sin(phi) - m3 * g * d * cos(phi))/A+((D*sin(lambda))/(b*A))*tan(delta)+d3+((B*v*sin(lambda))/(b*A))*tan(delta_d);

xdot=[xdot1 xdot2 xdot3];

== matlab function bike_model_yixiao/Physical Bike/Linear Bicycle Model with neglected fork angle (lambda=90deg, c=0) "THE SIMPLEST MODEL" ==
  data: states input; input input; xdot output; velocity input; disturbance input; parameters_real input; parameters_f_b_real input
function xdot = fcn(states,input,velocity,disturbance,parameters_real,parameters_f_b_real)

delta_d=input;
v=velocity;
d1=disturbance(1);
d2=disturbance(2);
d3=disturbance(3);

% 1=frame | 2=box
m1=parameters_f_b_real(1);
m2=parameters_f_b_real(2);
h1=parameters_f_b_real(3);
h2=parameters_f_b_real(4);
a1=parameters_f_b_real(5);
a2=parameters_f_b_real(6);
c1=parameters_f_b_real(7);
c2=parameters_f_b_real(8);
b1=parameters_f_b_real(9);
b2=parameters_f_b_real(10);
l1=parameters_f_b_real(11);
l2=parameters_f_b_real(12);

g=parameters_real(1);
%h=parameters_real(2);
b=parameters_real(3);
%a=parameters_real(4);
lambda=parameters_real(5);
c=parameters_real(6);

A=((m1/12)*((c1^2)+(b1^2)))+(m1*(h1^2))+((m2/12)*((c2^2)+(b2^2)))+(m2*(h2^2));
B=((m1/12)*((l1^2)+(b1^2)))-(m1*a1*h1)+((m2/12)*((c2^2)+(b2^2)))+(m2*a2*h2);
D=(((m1*h1)+(m2*h2))*(v^2))-(c*g*((m1*a1)-(m2*a2)));

phi=states(1);
delta=states(2);
phi_d=states(3);

xdot1=phi_d+d1;
xdot2=delta_d+d2;
xdot3=((((m1*h1)+(m2*h2))*g)/A)*phi+((D*sin(lambda))/(b*A))*delta+d3+((B*v*sin(lambda))/(b*A))*delta_d;

xdot=[xdot1 xdot2 xdot3];

== matlab function bike_model_yixiao/Global Angles and Coordinates Calculator - Velocity/Measured Bike Angles to Global Angles/MATLAB Function ==
  data: v input; parameters_model input; delta input; psi_d output; beta output
function [psi_d, beta]  = fcn(v, parameters_model, delta)

b = parameters_model(3);
a = parameters_model(4);

beta = atan((a / (b)) * tan(delta));
psi_d = (v / a) * sin(beta);

== matlab function bike_model_yixiao/Complementary filter/Roll Angle Estimation of Accelerometer/Lateral Acceleration Compensator/Linear Bicycle Model1 ==
  data: states input; input input; xdot output; velocity input; parameters_model input
function xdot = fcn(states,input,velocity,parameters_model)

delta_d=input;
v=velocity;

g=parameters_model(1);
h=parameters_model(2);
b=parameters_model(3);
a=parameters_model(4);
lambda=parameters_model(5);
c=parameters_model(6);

phi=states(1);
delta=states(2);
phi_d=states(3);

xdot1=phi_d;
xdot2=delta_d;
xdot3=(g/h)*phi+((a*v)/(b*h))*sin(lambda)*delta_d+((h*v^2-g*a*c)/(b*h^2))*sin(lambda)*delta;

xdot=[xdot1; xdot2; xdot3];

== matlab function bike_model_yixiao/Complementary filter/Roll Angle Estimation of Accelerometer/Lateral Acceleration Compensator/discrete ==
  data: states input; input input; x_next output; A input; B input
function x_next = fcn(states,input,A,B)





x_next=A*states+B*input;

== matlab function bike_model_yixiao/Balance Controller/MPC attempt 2/Reference States/Reference Roll Angle Calculator ==
  data: parameters_real input; velocity input; delta_ref input; phi_ref output
function phi_ref = fcn(parameters_real, velocity, delta_ref)
g = parameters_real(1);
b = parameters_real(3);
v = velocity;

phi_ref = -atan(v^2 / (g * b) * delta_ref); % tan(theta_ref));

== matlab function bike_model_yixiao/Balance Controller/MPC attempt 2/MATLAB Function1 ==
  data: x0 input size=3; u output; xk0 input size=6; u0 input size=1; Nc input size=1; Np input size=1; r input; Delta_t input; v input; eta output; xk output
function [u,eta,xk] =  mpc_Setpoint(x0,xk0,u0,Nc,Np,r,Delta_t,v)
% This Function export the Optimal MPC estimation based on the states
% It runs at timestep k (so now),calculate the signal input for next timestep.
% % % % % % % % % % % % % % % % % % % % % % % % % % % % % % % % % % % % % % 
% 
% Input: 
% -> x0 := The current(k_{th} step) states column (state-space model), includes
% [x0;y0;Psi0;u;v;w;]
% -> xk0 := The Augmented System states, includes [\delta x_m(k); y(k)]
% -> Nc := The control horizon, which means, take actions(manipulate the
% input signal in the next Nc steps)
% -> Np := Prediction Horizon,estimate the states in the next Np steps;ß
% -> r := The reference signal, indicating which states you want to
% achieve,[x_d;y_d;Psi_d;u_d;v_d;w_d;]; 
% -> Delta_t := The sample time for discritization
% % % % % % % % % % % % % % % % % % % % % % % % % % % % % % % % % % % % % % 
% 
% Output:
% -> eta := The optimal \delta U input signal for the system in next Nc Steps,
% [\delta_TauX1;\delta_TauY1;\delta_TauPsi1;\delta_TauX2;\delta_TauY2;...;TauXNc;TauYNc;TauPsiNc];
% -> xk  := The estimation of xk,which may be used for comparison how good
% it tracks the trajectory
 
%% Initialization





% u = zeros(3,1);



%%
[A_m,B_m] = Lin_Sys(v);

C_m = eye(3);
D_m = zeros(3,1);
% The Input Increment Setting

R_bar = zeros(Nc);

% The Input Weight setting
% 
K_u      = 10*eye(Nc,Nc);
for i = 1:Nc
   K_u(i,i) = 10;
end

K_bar = zeros(Np*3);
for i = 1:Np
   K_bar((3)*i-2,(3)*i-2) = 1e2; % The Weight for \Phi
   K_bar((3)*i-1,(3)*i-1) = 1e2; % The Weight for Steering \delta
   K_bar((3)*i,(3)*i)     = 1e3; % The Weight for \dot{\Phi}
end

K_bar((3)*i-2,(3)*i-2) = 10*K_bar((3)*i-2,(3)*i-2) ; % The terminal weight for \Phi
K_bar((3)*i-1,(3)*i-1) = 10*K_bar((3)*i-1,(3)*i-1) ; % The Terminal Weight for Steering \delta
K_bar((3)*i,(3)*i)     = 1000*K_bar((3)*i,(3)*i) ;  % The Terminal Weight for \dot{\Phi}
% Rs = ones(Np,3)*r;

% MagSurge = 400*1e4;
% MagSway  = 100*1e4;
% MagYaw   = 1e6*1e4;
% DeltaSurge = 5e4;
% DeltaSway  = 5e4;
% DeltaYaw   = 5e7;
% 
% MagSurge = 100*1e4;
% MagSway  = 100*1e4;
% MagYaw   = 1e6*1e4;
% DeltaSurge = 5e4;
% DeltaSway  = 5e4;
% DeltaYaw   = 5e7;
% MagSurge = 1e4;
% MagSway  = 1e4;
% MagYaw   = 1e4;
% 
% end


%% Discretization
coder.extrinsic('c2dm','sum');

Ap = zeros(3,3);
Bp = zeros(3,1);
Cp = zeros(3,3);
[Ap,Bp,Cp,~]=c2dm(A_m,B_m,C_m,D_m,Delta_t,'zoh');

%% Augumented System 
A_e = zeros(6,6);
B_e = zeros(6,1);
% Ce = zeros(3,6);

Phi_Phi = zeros(Nc,Nc);
Phi_R = zeros(Nc,Np);
Phi_F = zeros(Nc,6);
coder.extrinsic('mpcgain')
[Phi_Phi,Phi_F,Phi_R,A_e,B_e,~,~] = mpcgain(Ap,Bp,Cp,Nc,Np,r,K_bar);


%% solve the optimization problem

% H0 = 2*(Phi_Phi + R_bar); % 3*Nc by 3*Nc
% f0 = -2*(Phi_R-Phi_F*xk0); % 3*Nc by 1
% 
% 
% % The Positive Part for Manipulated Variable(Input) Constraints
% A_cons1 = eye(3*Nc,3*Nc);
% B_cons1 = zeros(3*Nc,1);
% for j = 1:Nc % The #column
%     for i = 1+j:Nc % The #row 
%     A_cons1(3*i-2:3*i,3*j-2:3*j) = eye(3);
% %     A_cons(3*(Nc+i)-2:3*(Nc+i),3*j-2:3*j) = -eye(3);
%     end
%     B_cons1(3*j-2:3*j,1) = [MagSurge;MagSway;MagYaw]-u0;
% %     B_cons(3*(Nc+i)-2:3*(Nc+i),1) =[10000*1e4;10000*1e4;1e4*1e5]+u0;
% end
% 
% % The Negative Part for Manipulated Variable(Input) Constraints
% A_cons2 = eye(3*Nc,3*Nc);
% B_cons2 = zeros(3*Nc,1);
% 
% for j = 1:Nc % The #column
%     for i = 1+j:Nc % The #row 
%     A_cons2(3*i-2:3*i,3*j-2:3*j) = -eye(3);
% %     A_cons2(3*(Nc+i)-2:3*(Nc+i),3*j-2:3*j) = -eye(3);
%     end
%     B_cons2(3*j-2:3*j,1) = [MagSurge;MagSway;MagYaw]+u0;
% %     B_cons2(3*(Nc+i)-2:3*(Nc+i),1) =[10000*1e4;10000*1e4;1e4*1e5]+u0;
% end
% 
% % The Constraints for Input Increment Positive Part
% 
% A_cons3 = eye(3*Nc,3*Nc);
% B_cons3 = zeros(3*Nc,1);
% 
% Wr = 1e3;  % The Multipiler for Increment Input
% 
% for i = 1:Nc % The #row
%     B_cons3(3*i-2:3*i,1) = [DeltaSurge;DeltaSway;DeltaYaw]*Wr;
% end
% 
% % The Constraints for Input Increment Negative Part
% 
% A_cons4 = -eye(3*Nc,3*Nc);
% B_cons4 = zeros(3*Nc,1);
% 
% for i = 1:Nc % The #row
%     B_cons4(3*i-2:3*i,1) = [DeltaSurge;DeltaSway;DeltaYaw]*Wr;
% end


% Constructing the 3Nc*3Nc Lower-Diagnol Identity Matrix P:
%      1     0     0     0     0     0     
%      0     1     0     0     0     0     
%      0     0     1     0     0     0     
%      1     0     0     1     0     0     
%      0     1     0     0     1     0     
%      0     0     1     0     0     1 3Nc*3Nc This is also useful for
%      constrainting the input U

% % The Input sequence as 
% % [ u0;u0;...]Nc*1
P = eye(Nc,Nc);
U0= zeros(Nc,1);
% 
% A_cons1 = zeros(Nc,Nc);
% B_cons1 = zeros(Nc,1);
% A_cons2 = zeros(Nc,Nc);
% B_cons2 = zeros(Nc,1);
% A_cons3 = eye(Nc,Nc);
% B_cons3 = zeros(Nc,1);
% A_cons4 = -eye(Nc,Nc);
% B_cons4 = zeros(Nc,1);
% 
% 
for j = 1:Nc % The #column
    for i = 1+j:Nc % The #row 
    P(i,j) = 1;
    end
    U0(j) = u0;
%     B_cons1(3*j-2:3*j,1) = [MagSurge;MagSway;MagYaw]-u0;
%     B_cons2(3*j-2:3*j,1) = [MagSurge;MagSway;MagYaw]+u0;
%     B_cons3(3*j-2:3*j,1) = [DeltaSurge;DeltaSway;DeltaYaw]*Wr;
end
% B_cons4 = B_cons3;
% A_cons1 = P;
% A_cons2 = -P;



H0 = 2*(Phi_Phi + R_bar+P.'*K_u*P); % Nc by Nc
f0 = 2*(-Phi_R+Phi_F*xk0+P.'*K_u*U0); % Nc by 1

% 
% A_cons = [A_cons1;A_cons2;A_cons3;A_cons4];
% B_cons = [B_cons1;B_cons2;B_cons3;B_cons4];
% 
% 
% A_cons = [A_cons1;A_cons2;];
% B_cons = [B_cons1;B_cons2;];

% B_cons1 = double(B_cons1);
x = zeros(Nc,1);
x=-H0\f0; % Calculate an Optimal Solution WITHOUT CONSTRAINTS
% x = QPhild(H0,f0,A_cons,B_cons);
% size(B_e)
% [x,fval] = quadprog(H0,f0,[],[],[],[]);
% [x,fval] = quadprog(H0,f0,A_cons,B_cons,A_Eq1,B_Eq1);
% coder.extrinsic('quadprog');
% x = quadprog(H0,f0,A_cons,B_cons);
eta = 0;
eta = x(1); % The force increments to be applied
u = u0 + eta;
xk = zeros(6,1);
xk = A_e*xk0 + B_e*eta;





function [A_m B_m] = Lin_Sys(v)

% % % % % % % % % % % % % % % % % % % % % % % % % % % % % % % % % % % 
% 3-DOF Ship model Linearization
% 
% Input:
% v : rear wheel velocity
%
% Output:
% A 3*3 Linearized System Matrix for \dot{x} = A x + B u
% B 3*1 The Coefficient Matrix for input u
% 
% 
% 
% state x:= [ \Phi \delta \dot{\Phi} ]
% % % % % % % % % % % % % % % % % % % % % % % % % % % % % % % % % % % 

persistent h_real b_real c_real lambda_real a_real g 
% Real Bike Parameters
% Global system (frame+box as 1 volume)
if isempty(h_real)
    h_real = 0.48;             % height of center of mass [m]
    b_real = 1.095;            % length between wheel centers [m]
    c_real = 0.06;             % length between front wheel contact point and the 
    lambda_real = deg2rad(70); % angle of the fork axis [deg]
    a_real = 0.34;             % b_real-0.77;
    g = 9.81;                  % gravity [m/s^2]
end

A_m = [0      0            1;
       0      0            0;
       g/h_real    sin(lambda_real)*(h_real*v^2-g*a_real*c_real)/(h_real^2*b_real)   0];
B_m = [0; 1; (a_real*v*sin(lambda_real))/(h_real*b_real)];
C_m = eye(3);
D_m = zeros(3,1);


 
% function [Phi_Phi,Phi_F,Phi_R,A_e, B_e,C_e,F,Phi] = mpcgain(Ap,Bp,Cp,Nc,Np,r,K_bar)
% 
% % coder.extrinsic('size','eye','zeros');
% % coder.varsize('m1',[]   );
% m1 = 0;
% n1 = 0;
% v = 0;
% wid = 0
% Phi_Phi = zeros(Nc,Nc);
% Phi_R = zeros(Nc,Np)
% 
% m1=size(Cp,1);
% [n1,n_in]=size(Bp);
% A_e=eye(n1+m1,n1+m1);
% A_e(1:n1,1:n1)=Ap;
% A_e(n1+1:n1+m1,1:n1)=Cp*Ap;
% B_e=zeros(n1+m1,n_in);
% B_e(1:n1,:)=Bp;
% B_e(n1+1:n1+m1,:)=Cp*Bp;
% C_e=zeros(m1,n1+m1);
% C_e(:,n1+1:n1+m1)=eye(m1,m1);
% [wid,~] = size(C_e);
% h = zeros(3*Np,6);
% F = zeros(3*Np,6);
% h(1:wid,:)=C_e;
% F(1:wid,:)=C_e*A_e;
% 
% for kk=2:Np
% h((kk-1)*wid+1:kk*wid,:)=h((kk-2)*wid+1:(kk-1)*wid,:)*A_e;
% F((kk-1)*wid+1:kk*wid,:)= F((kk-2)*wid+1:(kk-1)*wid,:)*A_e;
% end
% 
% v=h*B_e;
% 
% len1 = size(B_e,2);
% Phi=zeros(Np*wid,Nc*len1); %declare the dimension of Phi
% 
% Phi(:,1:len1)=v; % first column of Phi
% % len1 = wid; % the length for CB,CAB,...
% for i=2:Nc
%     Phi(:,(i-1)*len1+1:i*len1)=[zeros((i-1)*wid,len1);v(1:(Np-i+1)*wid,1:len1)]; %Toeplitz matrix
% end
% 
% BarRs = zeros(Np*wid,1);
% 
%     for i = 1:Np
%         BarRs((i-1)*wid+1:i*wid,1) = r;
%     end
% 
% % BarRs
% Phi_Phi = Phi.'*K_bar*Phi;
% Phi_Phi = (Phi_Phi.' + Phi_Phi)/2;
% % F
% Phi_F= Phi'*K_bar*F;
% Phi_R=Phi.'*K_bar*BarRs;
% 
% 
% 
%

== matlab function bike_model_yixiao/Balance Controller/MPC attempt 2/MATLAB Function2 ==
  data: u input; y output
function y = fcn(u)
coder.extrinsic('print')
print(u)
print(size(u))
y = size(u,1);
